simulink model "ESC_Tuning_Motors"  (R2024a)
settings: Solver=FixedStepAuto  StartTime=0.0  StopTime=inf  FixedStep=0.02  RelTol=1e-3  EnableMultiTasking=on
libraries: bbblueActuatorLib x4
settings Model: ExtModeTrigDuration=100  Creator=eduar  LastModifiedBy=eduar
settings SolverCC: PositivePriorityOrder=on
settings OptimizationCC: EnhancedBackFolding=on  PassReuseOutputArgsAs=Individual arguments  ZeroExternalMemoryAtStartup=off  ZeroInternalMemoryAtStartup=off  MaxStackSize=64  OptimizeBlockOrder=speed  DifferentSizesBufferReuse=on  OptimizationCustomize=off  EfficientTunableParamExpr=on
settings DebuggingCC: ParameterTunabilityLossMsg=error
settings HardwareCC: ProdBitPerPointer=32  ProdBitPerSizeT=32  ProdBitPerPtrDiffT=32  ProdLargestAtomicInteger=Long  ProdLargestAtomicFloat=Double  ProdWordSize=32  ProdHWDeviceType=ARM Compatible->ARM Cortex
settings SFSimCC: MATLABDynamicMemAlloc=off
settings RTWCC: Description=Embedded Coder  SystemTargetFile=ert.tlc  HardwareBoard=BeagleBone Blue  TLCOptions="-aInlineSetEventsForThisBaseRateFcn=TLC_FALSE -aSuppressMultiTaskScheduler=TLC_FALSE  -aRateBasedStepFcn=0"  TemplateMakefile=ert_default_tmf  Toolchain=GNU GCC BeagleBone Blue
settings CodeAppCC: ForceParamTrailComments=on  IgnoreCustomStorageClasses=off  OperatorAnnotations=on  SimulinkDataObjDesc=on  SFDataObjDesc=on  InsertBlockDesc=on
settings ERTTargetCC: SupportVariableSizeSignals=on

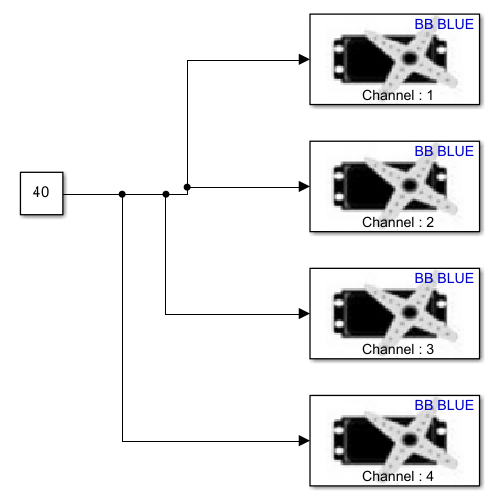
[thumbnail: Simulink's stored preview of the top-level diagram]
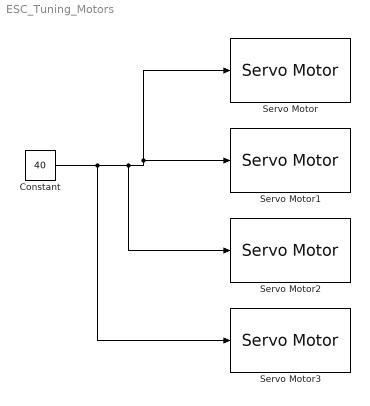
== system ESC_Tuning_Motors ==
  Constant : Constant  Value=40
  Servo Motor : bbblueActuatorLib/Servo Motor  channel=1  SimulateUsing=Code generation
  Servo Motor1 : bbblueActuatorLib/Servo Motor  channel=2  SimulateUsing=Code generation
  Servo Motor2 : bbblueActuatorLib/Servo Motor  channel=3  SimulateUsing=Code generation
  Servo Motor3 : bbblueActuatorLib/Servo Motor  channel=4  SimulateUsing=Code generation
  wires:
  Constant/1 -> Servo Motor3/1, Servo Motor2/1, Servo Motor/1, Servo Motor1/1
